simulink model "task_2_alpha05_mu_x"  (R2021b)
settings: Solver=FixedStepAuto  StartTime=0.0  StopTime=10  FixedStep=0.00005  RelTol=1e-3
settings Model: Creator=den  LastModifiedBy=den

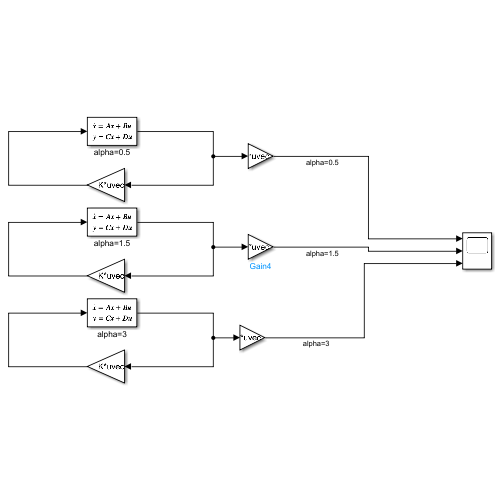
[thumbnail: Simulink's stored preview of the top-level diagram]
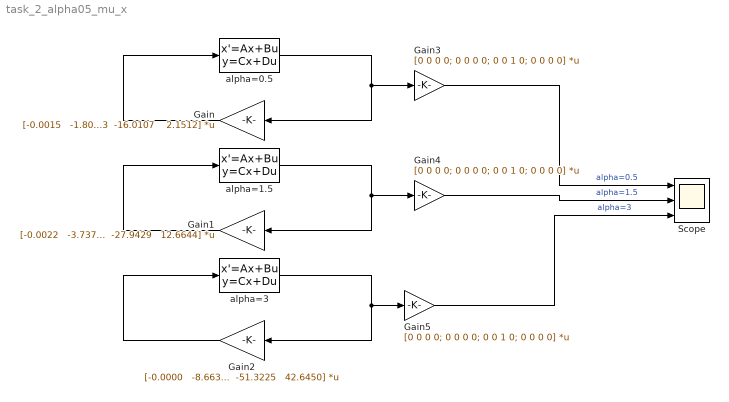
== system task_2_alpha05_mu_x ==
  Gain : Gain  Gain="[-0.0015   -1.8073  -16.0107    2.1512]"  Multiplication=Matrix(K*u) (u vector)
  Gain1 : Gain  Gain="[-0.0022   -3.7378  -27.9429   12.6644]"  Multiplication=Matrix(K*u) (u vector)
  Gain2 : Gain  Gain="[-0.0000   -8.6636  -51.3225   42.6450]"  Multiplication=Matrix(K*u) (u vector)
  Gain3 : Gain  Gain=[0 0 0 0; 0 0 0 0; 0 0 1 0; 0 0 0 0]  Multiplication=Matrix(K*u) (u vector)
  Gain4 : Gain  Gain=[0 0 0 0; 0 0 0 0; 0 0 1 0; 0 0 0 0]  Multiplication=Matrix(K*u) (u vector)
  Gain5 : Gain  Gain=[0 0 0 0; 0 0 0 0; 0 0 1 0; 0 0 0 0]  Multiplication=Matrix(K*u) (u vector)
  Scope : Scope  NumInputPorts=3
  alpha=0.5 : StateSpace  A=[-3 0 0 0; 0 3 0 0; 0 0 3 3; 0 0 -3 3]  B=[0; 7; 0; 1]  C=[1 0 0 0; 0 1 0 0; 0 0 1 0; 0 0 0 1]  D=[0; 0; 0; 0]  InitialCondition=[-3; 17; 2; -8]
  alpha=1.5 : StateSpace  A=[-3 0 0 0; 0 3 0 0; 0 0 3 3; 0 0 -3 3]  B=[0; 7; 0; 1]  C=[1 0 0 0; 0 1 0 0; 0 0 1 0; 0 0 0 1]  D=[0; 0; 0; 0]  InitialCondition=[-3; 17; 2; -8]
  alpha=3 : StateSpace  A=[-3 0 0 0; 0 3 0 0; 0 0 3 3; 0 0 -3 3]  B=[0; 7; 0; 1]  C=[1 0 0 0; 0 1 0 0; 0 0 1 0; 0 0 0 1]  D=[0; 0; 0; 0]  InitialCondition=[-3; 17; 2; -8]
  wires:
  Gain/1 -> alpha=0.5/1
  Gain1/1 -> alpha=1.5/1
  Gain2/1 -> alpha=3/1
  alpha=3/1 -> Gain2/1, Gain5/1
  alpha=0.5/1 -> Gain3/1, Gain/1
  alpha=1.5/1 -> Gain4/1, Gain1/1
  Gain3/1 -> Scope/1  "alpha=0.5"
  Gain4/1 -> Scope/2  "alpha=1.5"
  Gain5/1 -> Scope/3  "alpha=3"
